simulink model "multiplier"  (Simulink 8.0)
settings: Solver=VariableStepDiscrete  StartTime=0.0  StopTime=50  RelTol=1e-3
settings Model: Creator=dell  LastModifiedBy=dell
settings DebuggingCC: FcnCallInpInsideContextMsg=EnableAllAsWarning

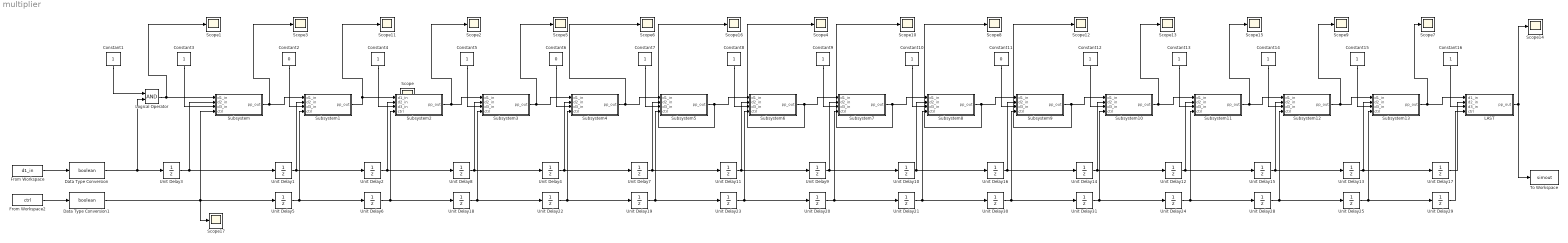
== system multiplier ==
  Constant{1,3..5,7..10,12..16} (13 alike) : Constant  OutDataTypeStr=boolean
  Constant11 : Constant  Value=0  OutDataTypeStr=boolean
  Constant2 : Constant  Value=0  OutDataTypeStr=boolean
  Constant6 : Constant  Value=0  OutDataTypeStr=boolean
  Data Type Conversion : DataTypeConversion  OutDataTypeStr=boolean
  Data Type Conversion1 : DataTypeConversion  OutDataTypeStr=boolean
  From Workspace : FromWorkspace  VariableName=d1_in  SampleTime=1
  From Workspace2 : FromWorkspace  VariableName=ctrl  SampleTime=1
  LAST : Subsystem
  Logical Operator : Logic  AllPortsSameDT=off  OutDataTypeStr=boolean
  Scope{,1..17} (18 alike) : Scope
      Scope10 settings: SaveName=ScopeData10
      Scope11 settings: SaveName=ScopeData11
      Scope12 settings: SaveName=ScopeData12
      Scope13 settings: SaveName=ScopeData13
      Scope14 settings: SaveName=ScopeData14
      Scope15 settings: SaveName=ScopeData15
      Scope16 settings: SaveName=ScopeData16
      Scope17 settings: SaveName=ScopeData17
      Scope2 settings: SaveName=ScopeData2
      Scope3 settings: SaveName=ScopeData3
      Scope4 settings: SaveName=ScopeData4
      Scope5 settings: SaveName=ScopeData5
      Scope6 settings: SaveName=ScopeData6
      Scope7 settings: SaveName=ScopeData7
      Scope8 settings: SaveName=ScopeData8
      Scope9 settings: SaveName=ScopeData9
  Subsystem : Subsystem
  Subsystem1 : Subsystem
  Subsystem10 : Subsystem
  Subsystem11 : Subsystem
  Subsystem12 : Subsystem
  Subsystem13 : Subsystem
  Subsystem2 : Subsystem
  Subsystem3 : Subsystem
  Subsystem4 : Subsystem
  Subsystem5 : Subsystem
  Subsystem6 : Subsystem
  Subsystem7 : Subsystem
  Subsystem8 : Subsystem
  Subsystem9 : Subsystem
  To Workspace : ToWorkspace  VariableName=simout  SampleTime=-1  SaveFormat=Timeseries
  Unit Delay{1..25,28..31} (29 alike) : UnitDelay
  wires:
  From Workspace/1 -> Data Type Conversion/1
  Logical Operator/1 -> Scope1/1, Subsystem/1(d1_in)
  Unit Delay3/1 -> Unit Delay1/1, Subsystem/2(d2_in)
  Subsystem/1(pp_out) -> Scope3/1, Subsystem1/1(d1_in)
  Subsystem1/1(pp_out) -> Scope11/1, Subsystem2/1(d1_in)
  Unit Delay5/1 -> Subsystem1/4(ctrl), Unit Delay6/1
  Constant1/1 -> Logical Operator/1
  Constant3/1 -> Subsystem/3(d3_in)
  Constant2/1 -> Subsystem1/3(d3_in)
  Constant4/1 -> Subsystem2/3(d3_in)
  From Workspace2/1 -> Data Type Conversion1/1
  Unit Delay1/1 -> Subsystem1/2(d2_in), Unit Delay2/1
  Unit Delay2/1 -> Subsystem2/2(d2_in), Unit Delay8/1
  Unit Delay8/1 -> Subsystem3/2(d2_in), Unit Delay4/1
  Unit Delay4/1 -> Subsystem4/2(d2_in), Unit Delay7/1
  Unit Delay7/1 -> Subsystem5/2(d2_in), Unit Delay11/1
  Unit Delay11/1 -> Subsystem6/2(d2_in), Unit Delay9/1
  Unit Delay9/1 -> Subsystem7/2(d2_in), Unit Delay10/1
  Unit Delay10/1 -> Subsystem8/2(d2_in), Unit Delay16/1
  Unit Delay16/1 -> Subsystem9/2(d2_in), Unit Delay14/1
  Unit Delay14/1 -> Subsystem10/2(d2_in), Unit Delay12/1
  Unit Delay12/1 -> Subsystem11/2(d2_in), Unit Delay15/1
  Unit Delay15/1 -> Subsystem12/2(d2_in), Unit Delay13/1
  Unit Delay13/1 -> Subsystem13/2(d2_in), Unit Delay17/1
  Unit Delay6/1 -> Subsystem2/4(ctrl), Unit Delay18/1
  Unit Delay18/1 -> Subsystem3/4(ctrl), Unit Delay22/1
  Unit Delay22/1 -> Subsystem4/4(ctrl), Unit Delay19/1
  Unit Delay19/1 -> Subsystem5/4(ctrl), Unit Delay23/1
  Unit Delay23/1 -> Subsystem6/4(ctrl), Unit Delay20/1
  Unit Delay20/1 -> Subsystem7/4(ctrl), Unit Delay21/1
  Unit Delay21/1 -> Subsystem8/4(ctrl), Unit Delay30/1
  Unit Delay30/1 -> Subsystem9/4(ctrl), Unit Delay31/1
  Unit Delay31/1 -> Subsystem10/4(ctrl), Unit Delay24/1
  Unit Delay24/1 -> Subsystem11/4(ctrl), Unit Delay28/1
  Unit Delay28/1 -> Subsystem12/4(ctrl), Unit Delay25/1
  Unit Delay25/1 -> Subsystem13/4(ctrl), Unit Delay29/1
  Subsystem2/1(pp_out) -> Scope2/1, Subsystem3/1(d1_in)
  Subsystem3/1(pp_out) -> Scope5/1, Subsystem4/1(d1_in)
  Subsystem4/1(pp_out) -> Scope6/1, Subsystem5/1(d1_in)
  Subsystem5/1(pp_out) -> Scope16/1, Subsystem6/1(d1_in)
  Subsystem6/1(pp_out) -> Scope4/1, Subsystem7/1(d1_in)
  Subsystem7/1(pp_out) -> Scope10/1, Subsystem8/1(d1_in)
  Subsystem8/1(pp_out) -> Scope8/1, Subsystem9/1(d1_in)
  Subsystem9/1(pp_out) -> Scope12/1, Subsystem10/1(d1_in)
  Subsystem10/1(pp_out) -> Scope13/1, Subsystem11/1(d1_in)
  Subsystem11/1(pp_out) -> Scope15/1, Subsystem12/1(d1_in)
  Subsystem12/1(pp_out) -> Scope9/1, Subsystem13/1(d1_in)
  Subsystem13/1(pp_out) -> Scope7/1, LAST/1(d1_in)
  Unit Delay17/1 -> LAST/2(d2_in)
  Unit Delay29/1 -> LAST/4(ctrl)
  Constant5/1 -> Subsystem3/3(d3_in)
  Constant6/1 -> Subsystem4/3(d3_in)
  Constant7/1 -> Subsystem5/3(d3_in)
  Constant8/1 -> Subsystem6/3(d3_in)
  Constant9/1 -> Subsystem7/3(d3_in)
  Constant10/1 -> Subsystem8/3(d3_in)
  Constant11/1 -> Subsystem9/3(d3_in)
  Constant12/1 -> Subsystem10/3(d3_in)
  Constant13/1 -> Subsystem11/3(d3_in)
  Constant14/1 -> Subsystem12/3(d3_in)
  Constant15/1 -> Subsystem13/3(d3_in)
  Constant16/1 -> LAST/3(d3_in)
  LAST/1(pp_out) -> Scope14/1, To Workspace/1
  Data Type Conversion/1 -> Logical Operator/2, Unit Delay3/1
  Data Type Conversion1/1 -> Scope17/1, Subsystem/4(ctrl), Unit Delay5/1

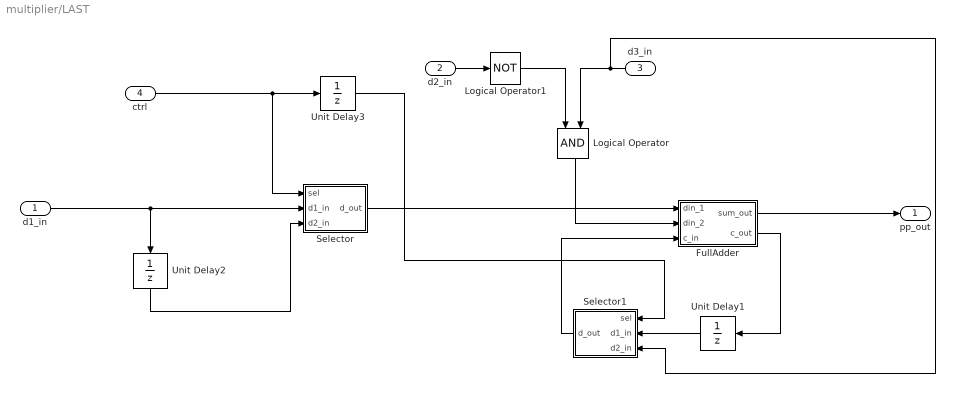
== system multiplier/LAST ==
  d1_in : Inport
  d2_in : Inport  Port=2
  d3_in : Inport  Port=3
  ctrl : Inport  Port=4
  FullAdder : Subsystem
  Logical Operator : Logic  AllPortsSameDT=off  OutDataTypeStr=boolean
  Logical Operator1 : Logic  Operator=NOT  AllPortsSameDT=off  OutDataTypeStr=boolean
  Selector : Subsystem
  Selector1 : Subsystem
  Unit Delay1 : UnitDelay
  Unit Delay2 : UnitDelay
  Unit Delay3 : UnitDelay
  pp_out : Outport
  wires:
  FullAdder/2(c_out) -> Unit Delay1/1
  d3_in/1 -> Logical Operator/2, Selector1/3(d2_in)
  ctrl/1 -> Unit Delay3/1, Selector/1(sel)
  d1_in/1 -> Selector/2(d1_in), Unit Delay2/1
  Unit Delay2/1 -> Selector/3(d2_in)
  d2_in/1 -> Logical Operator1/1
  Logical Operator/1 -> FullAdder/2(din_2)
  Selector/1(d_out) -> FullAdder/1(din_1)
  FullAdder/1(sum_out) -> pp_out/1
  Unit Delay1/1 -> Selector1/2(d1_in)
  Unit Delay3/1 -> Selector1/1(sel)
  Selector1/1(d_out) -> FullAdder/3(c_in)
  Logical Operator1/1 -> Logical Operator/1

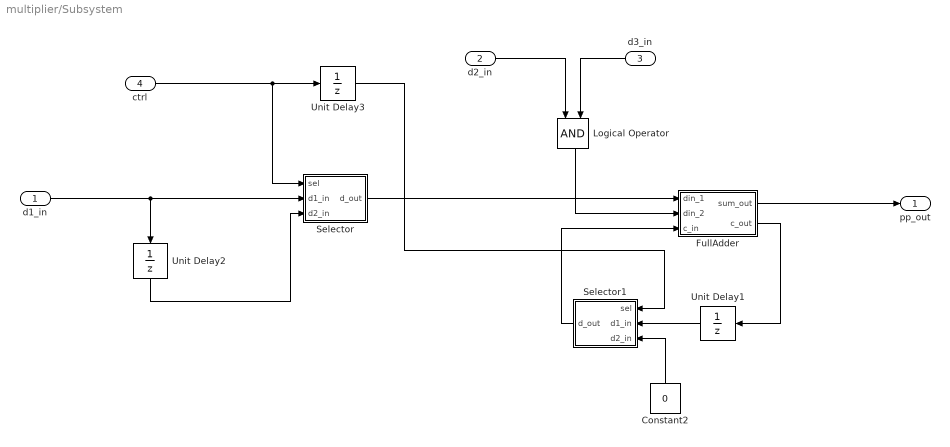
== system multiplier/Subsystem ==
  d1_in : Inport
  d2_in : Inport  Port=2
  d3_in : Inport  Port=3
  ctrl : Inport  Port=4
  Constant2 : Constant  Value=0  OutDataTypeStr=boolean
  FullAdder : Subsystem
  Logical Operator : Logic  AllPortsSameDT=off  OutDataTypeStr=boolean
  Selector : Subsystem
  Selector1 : Subsystem
  Unit Delay1 : UnitDelay
  Unit Delay2 : UnitDelay
  Unit Delay3 : UnitDelay
  pp_out : Outport
  wires:
  FullAdder/2(c_out) -> Unit Delay1/1
  d3_in/1 -> Logical Operator/2
  ctrl/1 -> Unit Delay3/1, Selector/1(sel)
  d1_in/1 -> Selector/2(d1_in), Unit Delay2/1
  Unit Delay2/1 -> Selector/3(d2_in)
  d2_in/1 -> Logical Operator/1
  Logical Operator/1 -> FullAdder/2(din_2)
  Selector/1(d_out) -> FullAdder/1(din_1)
  FullAdder/1(sum_out) -> pp_out/1
  Unit Delay1/1 -> Selector1/2(d1_in)
  Constant2/1 -> Selector1/3(d2_in)
  Unit Delay3/1 -> Selector1/1(sel)
  Selector1/1(d_out) -> FullAdder/3(c_in)

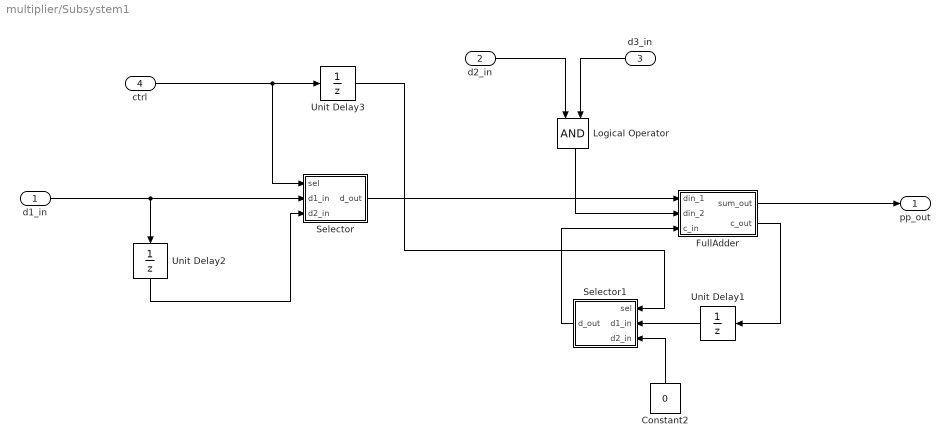
== system multiplier/Subsystem1 ==
  d1_in : Inport
  d2_in : Inport  Port=2
  d3_in : Inport  Port=3
  ctrl : Inport  Port=4
  Constant2 : Constant  Value=0  OutDataTypeStr=boolean
  FullAdder : Subsystem
  Logical Operator : Logic  AllPortsSameDT=off  OutDataTypeStr=boolean
  Selector : Subsystem
  Selector1 : Subsystem
  Unit Delay1 : UnitDelay
  Unit Delay2 : UnitDelay
  Unit Delay3 : UnitDelay
  pp_out : Outport
  wires:
  FullAdder/2(c_out) -> Unit Delay1/1
  d3_in/1 -> Logical Operator/2
  ctrl/1 -> Unit Delay3/1, Selector/1(sel)
  d1_in/1 -> Selector/2(d1_in), Unit Delay2/1
  Unit Delay2/1 -> Selector/3(d2_in)
  d2_in/1 -> Logical Operator/1
  Logical Operator/1 -> FullAdder/2(din_2)
  Selector/1(d_out) -> FullAdder/1(din_1)
  FullAdder/1(sum_out) -> pp_out/1
  Unit Delay1/1 -> Selector1/2(d1_in)
  Constant2/1 -> Selector1/3(d2_in)
  Unit Delay3/1 -> Selector1/1(sel)
  Selector1/1(d_out) -> FullAdder/3(c_in)

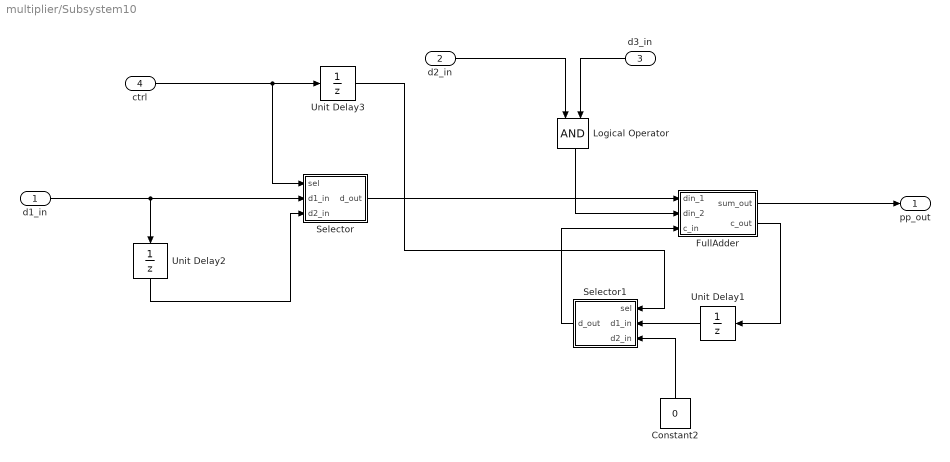
== system multiplier/Subsystem10 ==
  d1_in : Inport
  d2_in : Inport  Port=2
  d3_in : Inport  Port=3
  ctrl : Inport  Port=4
  Constant2 : Constant  Value=0  OutDataTypeStr=boolean
  FullAdder : Subsystem
  Logical Operator : Logic  AllPortsSameDT=off  OutDataTypeStr=boolean
  Selector : Subsystem
  Selector1 : Subsystem
  Unit Delay1 : UnitDelay
  Unit Delay2 : UnitDelay
  Unit Delay3 : UnitDelay
  pp_out : Outport
  wires:
  FullAdder/2(c_out) -> Unit Delay1/1
  d3_in/1 -> Logical Operator/2
  ctrl/1 -> Unit Delay3/1, Selector/1(sel)
  d1_in/1 -> Selector/2(d1_in), Unit Delay2/1
  Unit Delay2/1 -> Selector/3(d2_in)
  Logical Operator/1 -> FullAdder/2(din_2)
  Selector/1(d_out) -> FullAdder/1(din_1)
  FullAdder/1(sum_out) -> pp_out/1
  Unit Delay1/1 -> Selector1/2(d1_in)
  Unit Delay3/1 -> Selector1/1(sel)
  Selector1/1(d_out) -> FullAdder/3(c_in)
  d2_in/1 -> Logical Operator/1
  Constant2/1 -> Selector1/3(d2_in)

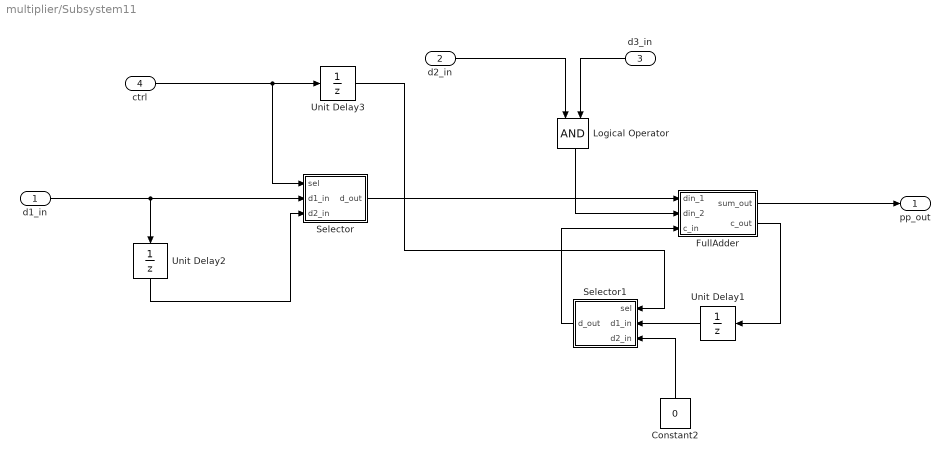
== system multiplier/Subsystem11 ==
  d1_in : Inport
  d2_in : Inport  Port=2
  d3_in : Inport  Port=3
  ctrl : Inport  Port=4
  Constant2 : Constant  Value=0  OutDataTypeStr=boolean
  FullAdder : Subsystem
  Logical Operator : Logic  AllPortsSameDT=off  OutDataTypeStr=boolean
  Selector : Subsystem
  Selector1 : Subsystem
  Unit Delay1 : UnitDelay
  Unit Delay2 : UnitDelay
  Unit Delay3 : UnitDelay
  pp_out : Outport
  wires:
  FullAdder/2(c_out) -> Unit Delay1/1
  d3_in/1 -> Logical Operator/2
  ctrl/1 -> Unit Delay3/1, Selector/1(sel)
  d1_in/1 -> Selector/2(d1_in), Unit Delay2/1
  Unit Delay2/1 -> Selector/3(d2_in)
  Logical Operator/1 -> FullAdder/2(din_2)
  Selector/1(d_out) -> FullAdder/1(din_1)
  FullAdder/1(sum_out) -> pp_out/1
  Unit Delay1/1 -> Selector1/2(d1_in)
  Unit Delay3/1 -> Selector1/1(sel)
  Selector1/1(d_out) -> FullAdder/3(c_in)
  d2_in/1 -> Logical Operator/1
  Constant2/1 -> Selector1/3(d2_in)

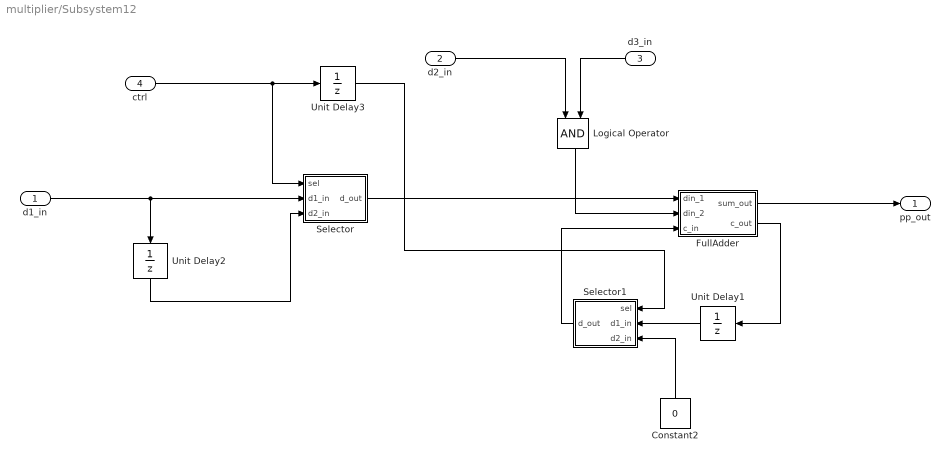
== system multiplier/Subsystem12 ==
  d1_in : Inport
  d2_in : Inport  Port=2
  d3_in : Inport  Port=3
  ctrl : Inport  Port=4
  Constant2 : Constant  Value=0  OutDataTypeStr=boolean
  FullAdder : Subsystem
  Logical Operator : Logic  AllPortsSameDT=off  OutDataTypeStr=boolean
  Selector : Subsystem
  Selector1 : Subsystem
  Unit Delay1 : UnitDelay
  Unit Delay2 : UnitDelay
  Unit Delay3 : UnitDelay
  pp_out : Outport
  wires:
  FullAdder/2(c_out) -> Unit Delay1/1
  d3_in/1 -> Logical Operator/2
  ctrl/1 -> Unit Delay3/1, Selector/1(sel)
  d1_in/1 -> Selector/2(d1_in), Unit Delay2/1
  Unit Delay2/1 -> Selector/3(d2_in)
  Logical Operator/1 -> FullAdder/2(din_2)
  Selector/1(d_out) -> FullAdder/1(din_1)
  FullAdder/1(sum_out) -> pp_out/1
  Unit Delay1/1 -> Selector1/2(d1_in)
  Unit Delay3/1 -> Selector1/1(sel)
  Selector1/1(d_out) -> FullAdder/3(c_in)
  d2_in/1 -> Logical Operator/1
  Constant2/1 -> Selector1/3(d2_in)

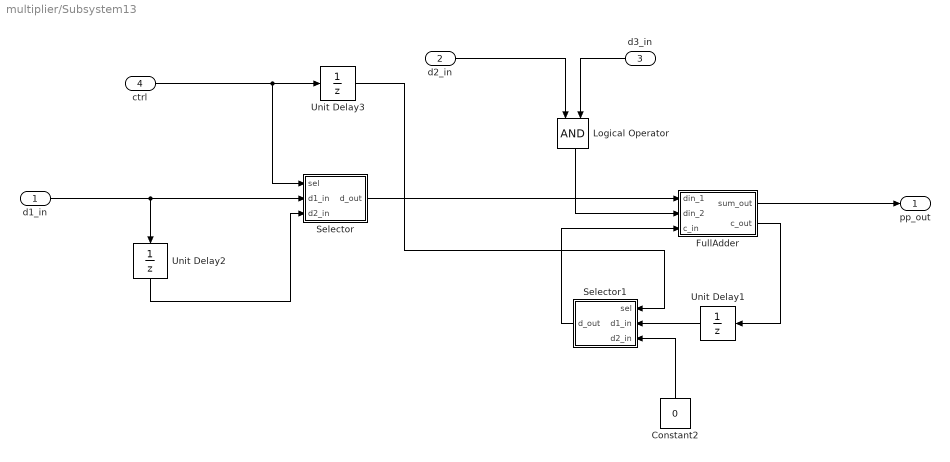
== system multiplier/Subsystem13 ==
  d1_in : Inport
  d2_in : Inport  Port=2
  d3_in : Inport  Port=3
  ctrl : Inport  Port=4
  Constant2 : Constant  Value=0  OutDataTypeStr=boolean
  FullAdder : Subsystem
  Logical Operator : Logic  AllPortsSameDT=off  OutDataTypeStr=boolean
  Selector : Subsystem
  Selector1 : Subsystem
  Unit Delay1 : UnitDelay
  Unit Delay2 : UnitDelay
  Unit Delay3 : UnitDelay
  pp_out : Outport
  wires:
  FullAdder/2(c_out) -> Unit Delay1/1
  d3_in/1 -> Logical Operator/2
  ctrl/1 -> Unit Delay3/1, Selector/1(sel)
  d1_in/1 -> Selector/2(d1_in), Unit Delay2/1
  Unit Delay2/1 -> Selector/3(d2_in)
  Logical Operator/1 -> FullAdder/2(din_2)
  Selector/1(d_out) -> FullAdder/1(din_1)
  FullAdder/1(sum_out) -> pp_out/1
  Unit Delay1/1 -> Selector1/2(d1_in)
  Unit Delay3/1 -> Selector1/1(sel)
  Selector1/1(d_out) -> FullAdder/3(c_in)
  d2_in/1 -> Logical Operator/1
  Constant2/1 -> Selector1/3(d2_in)

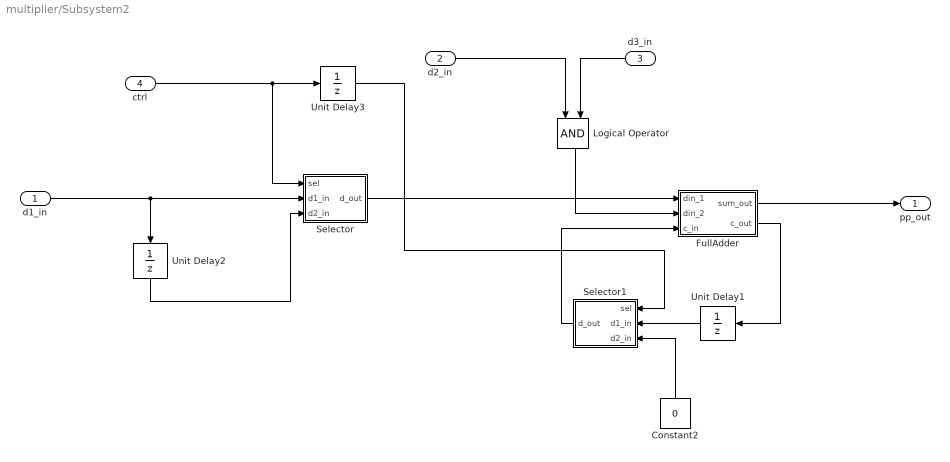
== system multiplier/Subsystem2 ==
  d1_in : Inport
  d2_in : Inport  Port=2
  d3_in : Inport  Port=3
  ctrl : Inport  Port=4
  Constant2 : Constant  Value=0  OutDataTypeStr=boolean
  FullAdder : Subsystem
  Logical Operator : Logic  AllPortsSameDT=off  OutDataTypeStr=boolean
  Selector : Subsystem
  Selector1 : Subsystem
  Unit Delay1 : UnitDelay
  Unit Delay2 : UnitDelay
  Unit Delay3 : UnitDelay
  pp_out : Outport
  wires:
  FullAdder/2(c_out) -> Unit Delay1/1
  d3_in/1 -> Logical Operator/2
  ctrl/1 -> Unit Delay3/1, Selector/1(sel)
  d1_in/1 -> Selector/2(d1_in), Unit Delay2/1
  Unit Delay2/1 -> Selector/3(d2_in)
  Logical Operator/1 -> FullAdder/2(din_2)
  Selector/1(d_out) -> FullAdder/1(din_1)
  FullAdder/1(sum_out) -> pp_out/1
  Unit Delay1/1 -> Selector1/2(d1_in)
  Unit Delay3/1 -> Selector1/1(sel)
  Selector1/1(d_out) -> FullAdder/3(c_in)
  d2_in/1 -> Logical Operator/1
  Constant2/1 -> Selector1/3(d2_in)

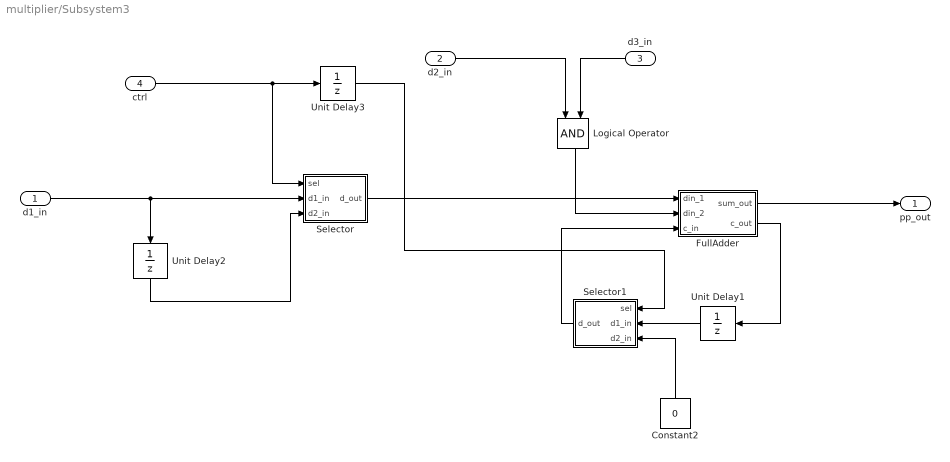
== system multiplier/Subsystem3 ==
  d1_in : Inport
  d2_in : Inport  Port=2
  d3_in : Inport  Port=3
  ctrl : Inport  Port=4
  Constant2 : Constant  Value=0  OutDataTypeStr=boolean
  FullAdder : Subsystem
  Logical Operator : Logic  AllPortsSameDT=off  OutDataTypeStr=boolean
  Selector : Subsystem
  Selector1 : Subsystem
  Unit Delay1 : UnitDelay
  Unit Delay2 : UnitDelay
  Unit Delay3 : UnitDelay
  pp_out : Outport
  wires:
  FullAdder/2(c_out) -> Unit Delay1/1
  d3_in/1 -> Logical Operator/2
  ctrl/1 -> Unit Delay3/1, Selector/1(sel)
  d1_in/1 -> Selector/2(d1_in), Unit Delay2/1
  Unit Delay2/1 -> Selector/3(d2_in)
  Logical Operator/1 -> FullAdder/2(din_2)
  Selector/1(d_out) -> FullAdder/1(din_1)
  FullAdder/1(sum_out) -> pp_out/1
  Unit Delay1/1 -> Selector1/2(d1_in)
  Unit Delay3/1 -> Selector1/1(sel)
  Selector1/1(d_out) -> FullAdder/3(c_in)
  d2_in/1 -> Logical Operator/1
  Constant2/1 -> Selector1/3(d2_in)

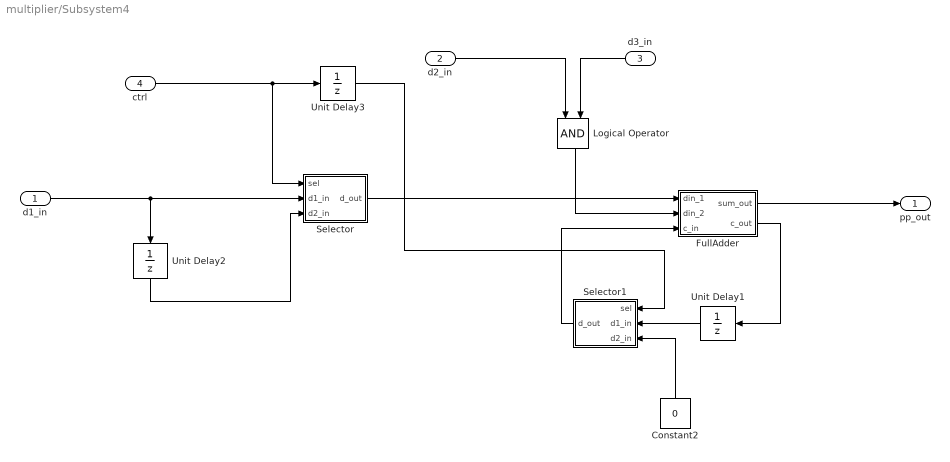
== system multiplier/Subsystem4 ==
  d1_in : Inport
  d2_in : Inport  Port=2
  d3_in : Inport  Port=3
  ctrl : Inport  Port=4
  Constant2 : Constant  Value=0  OutDataTypeStr=boolean
  FullAdder : Subsystem
  Logical Operator : Logic  AllPortsSameDT=off  OutDataTypeStr=boolean
  Selector : Subsystem
  Selector1 : Subsystem
  Unit Delay1 : UnitDelay
  Unit Delay2 : UnitDelay
  Unit Delay3 : UnitDelay
  pp_out : Outport
  wires:
  FullAdder/2(c_out) -> Unit Delay1/1
  d3_in/1 -> Logical Operator/2
  ctrl/1 -> Unit Delay3/1, Selector/1(sel)
  d1_in/1 -> Selector/2(d1_in), Unit Delay2/1
  Unit Delay2/1 -> Selector/3(d2_in)
  Logical Operator/1 -> FullAdder/2(din_2)
  Selector/1(d_out) -> FullAdder/1(din_1)
  FullAdder/1(sum_out) -> pp_out/1
  Unit Delay1/1 -> Selector1/2(d1_in)
  Unit Delay3/1 -> Selector1/1(sel)
  Selector1/1(d_out) -> FullAdder/3(c_in)
  d2_in/1 -> Logical Operator/1
  Constant2/1 -> Selector1/3(d2_in)

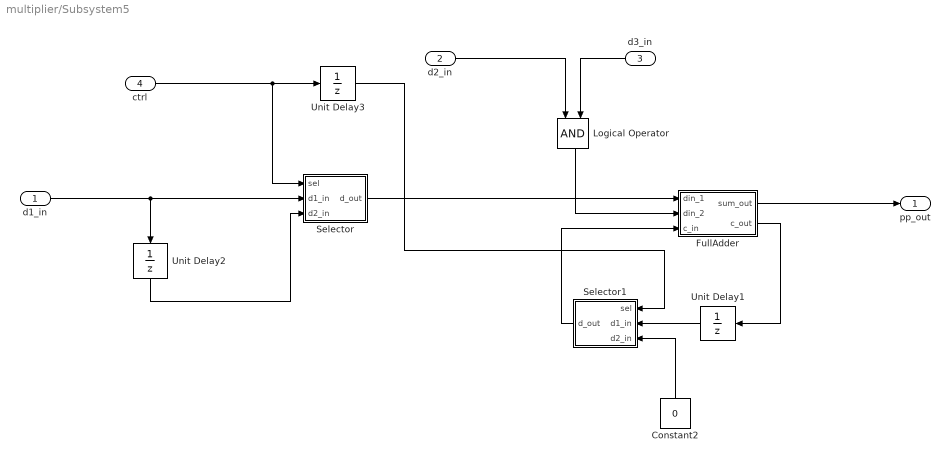
== system multiplier/Subsystem5 ==
  d1_in : Inport
  d2_in : Inport  Port=2
  d3_in : Inport  Port=3
  ctrl : Inport  Port=4
  Constant2 : Constant  Value=0  OutDataTypeStr=boolean
  FullAdder : Subsystem
  Logical Operator : Logic  AllPortsSameDT=off  OutDataTypeStr=boolean
  Selector : Subsystem
  Selector1 : Subsystem
  Unit Delay1 : UnitDelay
  Unit Delay2 : UnitDelay
  Unit Delay3 : UnitDelay
  pp_out : Outport
  wires:
  FullAdder/2(c_out) -> Unit Delay1/1
  d3_in/1 -> Logical Operator/2
  ctrl/1 -> Unit Delay3/1, Selector/1(sel)
  d1_in/1 -> Selector/2(d1_in), Unit Delay2/1
  Unit Delay2/1 -> Selector/3(d2_in)
  Logical Operator/1 -> FullAdder/2(din_2)
  Selector/1(d_out) -> FullAdder/1(din_1)
  FullAdder/1(sum_out) -> pp_out/1
  Unit Delay1/1 -> Selector1/2(d1_in)
  Unit Delay3/1 -> Selector1/1(sel)
  Selector1/1(d_out) -> FullAdder/3(c_in)
  d2_in/1 -> Logical Operator/1
  Constant2/1 -> Selector1/3(d2_in)

== system multiplier/Subsystem6 ==
  d1_in : Inport
  d2_in : Inport  Port=2
  d3_in : Inport  Port=3
  ctrl : Inport  Port=4
  Constant2 : Constant  Value=0  OutDataTypeStr=boolean
  FullAdder : Subsystem
  Logical Operator : Logic  AllPortsSameDT=off  OutDataTypeStr=boolean
  Selector : Subsystem
  Selector1 : Subsystem
  Unit Delay1 : UnitDelay
  Unit Delay2 : UnitDelay
  Unit Delay3 : UnitDelay
  pp_out : Outport
  wires:
  FullAdder/2(c_out) -> Unit Delay1/1
  d3_in/1 -> Logical Operator/2
  ctrl/1 -> Unit Delay3/1, Selector/1(sel)
  d1_in/1 -> Selector/2(d1_in), Unit Delay2/1
  Unit Delay2/1 -> Selector/3(d2_in)
  Logical Operator/1 -> FullAdder/2(din_2)
  Selector/1(d_out) -> FullAdder/1(din_1)
  FullAdder/1(sum_out) -> pp_out/1
  Unit Delay1/1 -> Selector1/2(d1_in)
  Unit Delay3/1 -> Selector1/1(sel)
  Selector1/1(d_out) -> FullAdder/3(c_in)
  d2_in/1 -> Logical Operator/1
  Constant2/1 -> Selector1/3(d2_in)

== system multiplier/Subsystem7 ==
  d1_in : Inport
  d2_in : Inport  Port=2
  d3_in : Inport  Port=3
  ctrl : Inport  Port=4
  Constant2 : Constant  Value=0  OutDataTypeStr=boolean
  FullAdder : Subsystem
  Logical Operator : Logic  AllPortsSameDT=off  OutDataTypeStr=boolean
  Selector : Subsystem
  Selector1 : Subsystem
  Unit Delay1 : UnitDelay
  Unit Delay2 : UnitDelay
  Unit Delay3 : UnitDelay
  pp_out : Outport
  wires:
  FullAdder/2(c_out) -> Unit Delay1/1
  d3_in/1 -> Logical Operator/2
  ctrl/1 -> Unit Delay3/1, Selector/1(sel)
  d1_in/1 -> Selector/2(d1_in), Unit Delay2/1
  Unit Delay2/1 -> Selector/3(d2_in)
  Logical Operator/1 -> FullAdder/2(din_2)
  Selector/1(d_out) -> FullAdder/1(din_1)
  FullAdder/1(sum_out) -> pp_out/1
  Unit Delay1/1 -> Selector1/2(d1_in)
  Unit Delay3/1 -> Selector1/1(sel)
  Selector1/1(d_out) -> FullAdder/3(c_in)
  d2_in/1 -> Logical Operator/1
  Constant2/1 -> Selector1/3(d2_in)

== system multiplier/Subsystem8 ==
  d1_in : Inport
  d2_in : Inport  Port=2
  d3_in : Inport  Port=3
  ctrl : Inport  Port=4
  Constant2 : Constant  Value=0  OutDataTypeStr=boolean
  FullAdder : Subsystem
  Logical Operator : Logic  AllPortsSameDT=off  OutDataTypeStr=boolean
  Selector : Subsystem
  Selector1 : Subsystem
  Unit Delay1 : UnitDelay
  Unit Delay2 : UnitDelay
  Unit Delay3 : UnitDelay
  pp_out : Outport
  wires:
  FullAdder/2(c_out) -> Unit Delay1/1
  d3_in/1 -> Logical Operator/2
  ctrl/1 -> Unit Delay3/1, Selector/1(sel)
  d1_in/1 -> Selector/2(d1_in), Unit Delay2/1
  Unit Delay2/1 -> Selector/3(d2_in)
  Logical Operator/1 -> FullAdder/2(din_2)
  Selector/1(d_out) -> FullAdder/1(din_1)
  FullAdder/1(sum_out) -> pp_out/1
  Unit Delay1/1 -> Selector1/2(d1_in)
  Unit Delay3/1 -> Selector1/1(sel)
  Selector1/1(d_out) -> FullAdder/3(c_in)
  d2_in/1 -> Logical Operator/1
  Constant2/1 -> Selector1/3(d2_in)

== system multiplier/Subsystem9 ==
  d1_in : Inport
  d2_in : Inport  Port=2
  d3_in : Inport  Port=3
  ctrl : Inport  Port=4
  Constant2 : Constant  Value=0  OutDataTypeStr=boolean
  FullAdder : Subsystem
  Logical Operator : Logic  AllPortsSameDT=off  OutDataTypeStr=boolean
  Selector : Subsystem
  Selector1 : Subsystem
  Unit Delay1 : UnitDelay
  Unit Delay2 : UnitDelay
  Unit Delay3 : UnitDelay
  pp_out : Outport
  wires:
  FullAdder/2(c_out) -> Unit Delay1/1
  d3_in/1 -> Logical Operator/2
  ctrl/1 -> Unit Delay3/1, Selector/1(sel)
  d1_in/1 -> Selector/2(d1_in), Unit Delay2/1
  Unit Delay2/1 -> Selector/3(d2_in)
  Logical Operator/1 -> FullAdder/2(din_2)
  Selector/1(d_out) -> FullAdder/1(din_1)
  FullAdder/1(sum_out) -> pp_out/1
  Unit Delay1/1 -> Selector1/2(d1_in)
  Unit Delay3/1 -> Selector1/1(sel)
  Selector1/1(d_out) -> FullAdder/3(c_in)
  d2_in/1 -> Logical Operator/1
  Constant2/1 -> Selector1/3(d2_in)

== system multiplier/LAST/FullAdder ==
  din_1 : Inport  OutDataTypeStr=boolean
  din_2 : Inport  Port=2  OutDataTypeStr=boolean
  c_in : Inport  Port=3  OutDataTypeStr=boolean
  Bus Creator : BusCreator  Inputs=3
  Combinatorial  Logic : CombinatorialLogic  TruthTable=[0;1;1;0;1;0;0;1]
  Combinatorial  Logic1 : CombinatorialLogic  TruthTable=[0;0;0;1;0;1;1;1]
  sum_out : Outport
  c_out : Outport  Port=2
  wires:
  Combinatorial  Logic/1 -> sum_out/1
  din_1/1 -> Bus Creator/1
  din_2/1 -> Bus Creator/2
  c_in/1 -> Bus Creator/3
  Bus Creator/1 -> Combinatorial  Logic/1, Combinatorial  Logic1/1
  Combinatorial  Logic1/1 -> c_out/1

== system multiplier/LAST/Selector ==
  sel : Inport
  d1_in : Inport  Port=2
  d2_in : Inport  Port=3
  Bus Creator : BusCreator  Inputs=3
  Combinatorial  Logic : CombinatorialLogic  TruthTable=[0;0;1;1;0;1;0;1]
  d_out : Outport
  wires:
  sel/1 -> Bus Creator/1
  d1_in/1 -> Bus Creator/2
  d2_in/1 -> Bus Creator/3
  Bus Creator/1 -> Combinatorial  Logic/1
  Combinatorial  Logic/1 -> d_out/1

== system multiplier/LAST/Selector1 ==
  sel : Inport
  d1_in : Inport  Port=2
  d2_in : Inport  Port=3
  Bus Creator : BusCreator  Inputs=3
  Combinatorial  Logic : CombinatorialLogic  TruthTable=[0;0;1;1;0;1;0;1]
  d_out : Outport
  wires:
  sel/1 -> Bus Creator/1
  d1_in/1 -> Bus Creator/2
  d2_in/1 -> Bus Creator/3
  Bus Creator/1 -> Combinatorial  Logic/1
  Combinatorial  Logic/1 -> d_out/1

== system multiplier/Subsystem/FullAdder ==
  din_1 : Inport  OutDataTypeStr=boolean
  din_2 : Inport  Port=2  OutDataTypeStr=boolean
  c_in : Inport  Port=3  OutDataTypeStr=boolean
  Bus Creator : BusCreator  Inputs=3
  Combinatorial  Logic : CombinatorialLogic  TruthTable=[0;1;1;0;1;0;0;1]
  Combinatorial  Logic1 : CombinatorialLogic  TruthTable=[0;0;0;1;0;1;1;1]
  sum_out : Outport
  c_out : Outport  Port=2
  wires:
  Combinatorial  Logic/1 -> sum_out/1
  din_1/1 -> Bus Creator/1
  din_2/1 -> Bus Creator/2
  c_in/1 -> Bus Creator/3
  Bus Creator/1 -> Combinatorial  Logic/1, Combinatorial  Logic1/1
  Combinatorial  Logic1/1 -> c_out/1

== system multiplier/Subsystem/Selector ==
  sel : Inport
  d1_in : Inport  Port=2
  d2_in : Inport  Port=3
  Bus Creator : BusCreator  Inputs=3
  Combinatorial  Logic : CombinatorialLogic  TruthTable=[0;0;1;1;0;1;0;1]
  d_out : Outport
  wires:
  sel/1 -> Bus Creator/1
  d1_in/1 -> Bus Creator/2
  d2_in/1 -> Bus Creator/3
  Bus Creator/1 -> Combinatorial  Logic/1
  Combinatorial  Logic/1 -> d_out/1

== system multiplier/Subsystem/Selector1 ==
  sel : Inport
  d1_in : Inport  Port=2
  d2_in : Inport  Port=3
  Bus Creator : BusCreator  Inputs=3
  Combinatorial  Logic : CombinatorialLogic  TruthTable=[0;0;1;1;0;1;0;1]
  d_out : Outport
  wires:
  sel/1 -> Bus Creator/1
  d1_in/1 -> Bus Creator/2
  d2_in/1 -> Bus Creator/3
  Bus Creator/1 -> Combinatorial  Logic/1
  Combinatorial  Logic/1 -> d_out/1

== system multiplier/Subsystem1/FullAdder ==
  din_1 : Inport  OutDataTypeStr=boolean
  din_2 : Inport  Port=2  OutDataTypeStr=boolean
  c_in : Inport  Port=3  OutDataTypeStr=boolean
  Bus Creator : BusCreator  Inputs=3
  Combinatorial  Logic : CombinatorialLogic  TruthTable=[0;1;1;0;1;0;0;1]
  Combinatorial  Logic1 : CombinatorialLogic  TruthTable=[0;0;0;1;0;1;1;1]
  sum_out : Outport
  c_out : Outport  Port=2
  wires:
  Combinatorial  Logic/1 -> sum_out/1
  din_1/1 -> Bus Creator/1
  din_2/1 -> Bus Creator/2
  c_in/1 -> Bus Creator/3
  Bus Creator/1 -> Combinatorial  Logic/1, Combinatorial  Logic1/1
  Combinatorial  Logic1/1 -> c_out/1

== system multiplier/Subsystem1/Selector ==
  sel : Inport
  d1_in : Inport  Port=2
  d2_in : Inport  Port=3
  Bus Creator : BusCreator  Inputs=3
  Combinatorial  Logic : CombinatorialLogic  TruthTable=[0;0;1;1;0;1;0;1]
  d_out : Outport
  wires:
  sel/1 -> Bus Creator/1
  d1_in/1 -> Bus Creator/2
  d2_in/1 -> Bus Creator/3
  Bus Creator/1 -> Combinatorial  Logic/1
  Combinatorial  Logic/1 -> d_out/1

== system multiplier/Subsystem1/Selector1 ==
  sel : Inport
  d1_in : Inport  Port=2
  d2_in : Inport  Port=3
  Bus Creator : BusCreator  Inputs=3
  Combinatorial  Logic : CombinatorialLogic  TruthTable=[0;0;1;1;0;1;0;1]
  d_out : Outport
  wires:
  sel/1 -> Bus Creator/1
  d1_in/1 -> Bus Creator/2
  d2_in/1 -> Bus Creator/3
  Bus Creator/1 -> Combinatorial  Logic/1
  Combinatorial  Logic/1 -> d_out/1

== system multiplier/Subsystem10/FullAdder ==
  din_1 : Inport  OutDataTypeStr=boolean
  din_2 : Inport  Port=2  OutDataTypeStr=boolean
  c_in : Inport  Port=3  OutDataTypeStr=boolean
  Bus Creator : BusCreator  Inputs=3
  Combinatorial  Logic : CombinatorialLogic  TruthTable=[0;1;1;0;1;0;0;1]
  Combinatorial  Logic1 : CombinatorialLogic  TruthTable=[0;0;0;1;0;1;1;1]
  sum_out : Outport
  c_out : Outport  Port=2
  wires:
  Combinatorial  Logic/1 -> sum_out/1
  din_1/1 -> Bus Creator/1
  din_2/1 -> Bus Creator/2
  c_in/1 -> Bus Creator/3
  Bus Creator/1 -> Combinatorial  Logic/1, Combinatorial  Logic1/1
  Combinatorial  Logic1/1 -> c_out/1

== system multiplier/Subsystem10/Selector ==
  sel : Inport
  d1_in : Inport  Port=2
  d2_in : Inport  Port=3
  Bus Creator : BusCreator  Inputs=3
  Combinatorial  Logic : CombinatorialLogic  TruthTable=[0;0;1;1;0;1;0;1]
  d_out : Outport
  wires:
  sel/1 -> Bus Creator/1
  d1_in/1 -> Bus Creator/2
  d2_in/1 -> Bus Creator/3
  Bus Creator/1 -> Combinatorial  Logic/1
  Combinatorial  Logic/1 -> d_out/1

== system multiplier/Subsystem10/Selector1 ==
  sel : Inport
  d1_in : Inport  Port=2
  d2_in : Inport  Port=3
  Bus Creator : BusCreator  Inputs=3
  Combinatorial  Logic : CombinatorialLogic  TruthTable=[0;0;1;1;0;1;0;1]
  d_out : Outport
  wires:
  sel/1 -> Bus Creator/1
  d1_in/1 -> Bus Creator/2
  d2_in/1 -> Bus Creator/3
  Bus Creator/1 -> Combinatorial  Logic/1
  Combinatorial  Logic/1 -> d_out/1

== system multiplier/Subsystem11/FullAdder ==
  din_1 : Inport  OutDataTypeStr=boolean
  din_2 : Inport  Port=2  OutDataTypeStr=boolean
  c_in : Inport  Port=3  OutDataTypeStr=boolean
  Bus Creator : BusCreator  Inputs=3
  Combinatorial  Logic : CombinatorialLogic  TruthTable=[0;1;1;0;1;0;0;1]
  Combinatorial  Logic1 : CombinatorialLogic  TruthTable=[0;0;0;1;0;1;1;1]
  sum_out : Outport
  c_out : Outport  Port=2
  wires:
  Combinatorial  Logic/1 -> sum_out/1
  din_1/1 -> Bus Creator/1
  din_2/1 -> Bus Creator/2
  c_in/1 -> Bus Creator/3
  Bus Creator/1 -> Combinatorial  Logic/1, Combinatorial  Logic1/1
  Combinatorial  Logic1/1 -> c_out/1

== system multiplier/Subsystem11/Selector ==
  sel : Inport
  d1_in : Inport  Port=2
  d2_in : Inport  Port=3
  Bus Creator : BusCreator  Inputs=3
  Combinatorial  Logic : CombinatorialLogic  TruthTable=[0;0;1;1;0;1;0;1]
  d_out : Outport
  wires:
  sel/1 -> Bus Creator/1
  d1_in/1 -> Bus Creator/2
  d2_in/1 -> Bus Creator/3
  Bus Creator/1 -> Combinatorial  Logic/1
  Combinatorial  Logic/1 -> d_out/1

== system multiplier/Subsystem11/Selector1 ==
  sel : Inport
  d1_in : Inport  Port=2
  d2_in : Inport  Port=3
  Bus Creator : BusCreator  Inputs=3
  Combinatorial  Logic : CombinatorialLogic  TruthTable=[0;0;1;1;0;1;0;1]
  d_out : Outport
  wires:
  sel/1 -> Bus Creator/1
  d1_in/1 -> Bus Creator/2
  d2_in/1 -> Bus Creator/3
  Bus Creator/1 -> Combinatorial  Logic/1
  Combinatorial  Logic/1 -> d_out/1

== system multiplier/Subsystem12/FullAdder ==
  din_1 : Inport  OutDataTypeStr=boolean
  din_2 : Inport  Port=2  OutDataTypeStr=boolean
  c_in : Inport  Port=3  OutDataTypeStr=boolean
  Bus Creator : BusCreator  Inputs=3
  Combinatorial  Logic : CombinatorialLogic  TruthTable=[0;1;1;0;1;0;0;1]
  Combinatorial  Logic1 : CombinatorialLogic  TruthTable=[0;0;0;1;0;1;1;1]
  sum_out : Outport
  c_out : Outport  Port=2
  wires:
  Combinatorial  Logic/1 -> sum_out/1
  din_1/1 -> Bus Creator/1
  din_2/1 -> Bus Creator/2
  c_in/1 -> Bus Creator/3
  Bus Creator/1 -> Combinatorial  Logic/1, Combinatorial  Logic1/1
  Combinatorial  Logic1/1 -> c_out/1

== system multiplier/Subsystem12/Selector ==
  sel : Inport
  d1_in : Inport  Port=2
  d2_in : Inport  Port=3
  Bus Creator : BusCreator  Inputs=3
  Combinatorial  Logic : CombinatorialLogic  TruthTable=[0;0;1;1;0;1;0;1]
  d_out : Outport
  wires:
  sel/1 -> Bus Creator/1
  d1_in/1 -> Bus Creator/2
  d2_in/1 -> Bus Creator/3
  Bus Creator/1 -> Combinatorial  Logic/1
  Combinatorial  Logic/1 -> d_out/1

== system multiplier/Subsystem12/Selector1 ==
  sel : Inport
  d1_in : Inport  Port=2
  d2_in : Inport  Port=3
  Bus Creator : BusCreator  Inputs=3
  Combinatorial  Logic : CombinatorialLogic  TruthTable=[0;0;1;1;0;1;0;1]
  d_out : Outport
  wires:
  sel/1 -> Bus Creator/1
  d1_in/1 -> Bus Creator/2
  d2_in/1 -> Bus Creator/3
  Bus Creator/1 -> Combinatorial  Logic/1
  Combinatorial  Logic/1 -> d_out/1

== system multiplier/Subsystem13/FullAdder ==
  din_1 : Inport  OutDataTypeStr=boolean
  din_2 : Inport  Port=2  OutDataTypeStr=boolean
  c_in : Inport  Port=3  OutDataTypeStr=boolean
  Bus Creator : BusCreator  Inputs=3
  Combinatorial  Logic : CombinatorialLogic  TruthTable=[0;1;1;0;1;0;0;1]
  Combinatorial  Logic1 : CombinatorialLogic  TruthTable=[0;0;0;1;0;1;1;1]
  sum_out : Outport
  c_out : Outport  Port=2
  wires:
  Combinatorial  Logic/1 -> sum_out/1
  din_1/1 -> Bus Creator/1
  din_2/1 -> Bus Creator/2
  c_in/1 -> Bus Creator/3
  Bus Creator/1 -> Combinatorial  Logic/1, Combinatorial  Logic1/1
  Combinatorial  Logic1/1 -> c_out/1

== system multiplier/Subsystem13/Selector ==
  sel : Inport
  d1_in : Inport  Port=2
  d2_in : Inport  Port=3
  Bus Creator : BusCreator  Inputs=3
  Combinatorial  Logic : CombinatorialLogic  TruthTable=[0;0;1;1;0;1;0;1]
  d_out : Outport
  wires:
  sel/1 -> Bus Creator/1
  d1_in/1 -> Bus Creator/2
  d2_in/1 -> Bus Creator/3
  Bus Creator/1 -> Combinatorial  Logic/1
  Combinatorial  Logic/1 -> d_out/1

== system multiplier/Subsystem13/Selector1 ==
  sel : Inport
  d1_in : Inport  Port=2
  d2_in : Inport  Port=3
  Bus Creator : BusCreator  Inputs=3
  Combinatorial  Logic : CombinatorialLogic  TruthTable=[0;0;1;1;0;1;0;1]
  d_out : Outport
  wires:
  sel/1 -> Bus Creator/1
  d1_in/1 -> Bus Creator/2
  d2_in/1 -> Bus Creator/3
  Bus Creator/1 -> Combinatorial  Logic/1
  Combinatorial  Logic/1 -> d_out/1

== system multiplier/Subsystem2/FullAdder ==
  din_1 : Inport  OutDataTypeStr=boolean
  din_2 : Inport  Port=2  OutDataTypeStr=boolean
  c_in : Inport  Port=3  OutDataTypeStr=boolean
  Bus Creator : BusCreator  Inputs=3
  Combinatorial  Logic : CombinatorialLogic  TruthTable=[0;1;1;0;1;0;0;1]
  Combinatorial  Logic1 : CombinatorialLogic  TruthTable=[0;0;0;1;0;1;1;1]
  sum_out : Outport
  c_out : Outport  Port=2
  wires:
  Combinatorial  Logic/1 -> sum_out/1
  din_1/1 -> Bus Creator/1
  din_2/1 -> Bus Creator/2
  c_in/1 -> Bus Creator/3
  Bus Creator/1 -> Combinatorial  Logic/1, Combinatorial  Logic1/1
  Combinatorial  Logic1/1 -> c_out/1

== system multiplier/Subsystem2/Selector ==
  sel : Inport
  d1_in : Inport  Port=2
  d2_in : Inport  Port=3
  Bus Creator : BusCreator  Inputs=3
  Combinatorial  Logic : CombinatorialLogic  TruthTable=[0;0;1;1;0;1;0;1]
  d_out : Outport
  wires:
  sel/1 -> Bus Creator/1
  d1_in/1 -> Bus Creator/2
  d2_in/1 -> Bus Creator/3
  Bus Creator/1 -> Combinatorial  Logic/1
  Combinatorial  Logic/1 -> d_out/1

== system multiplier/Subsystem2/Selector1 ==
  sel : Inport
  d1_in : Inport  Port=2
  d2_in : Inport  Port=3
  Bus Creator : BusCreator  Inputs=3
  Combinatorial  Logic : CombinatorialLogic  TruthTable=[0;0;1;1;0;1;0;1]
  d_out : Outport
  wires:
  sel/1 -> Bus Creator/1
  d1_in/1 -> Bus Creator/2
  d2_in/1 -> Bus Creator/3
  Bus Creator/1 -> Combinatorial  Logic/1
  Combinatorial  Logic/1 -> d_out/1

== system multiplier/Subsystem3/FullAdder ==
  din_1 : Inport  OutDataTypeStr=boolean
  din_2 : Inport  Port=2  OutDataTypeStr=boolean
  c_in : Inport  Port=3  OutDataTypeStr=boolean
  Bus Creator : BusCreator  Inputs=3
  Combinatorial  Logic : CombinatorialLogic  TruthTable=[0;1;1;0;1;0;0;1]
  Combinatorial  Logic1 : CombinatorialLogic  TruthTable=[0;0;0;1;0;1;1;1]
  sum_out : Outport
  c_out : Outport  Port=2
  wires:
  Combinatorial  Logic/1 -> sum_out/1
  din_1/1 -> Bus Creator/1
  din_2/1 -> Bus Creator/2
  c_in/1 -> Bus Creator/3
  Bus Creator/1 -> Combinatorial  Logic/1, Combinatorial  Logic1/1
  Combinatorial  Logic1/1 -> c_out/1

== system multiplier/Subsystem3/Selector ==
  sel : Inport
  d1_in : Inport  Port=2
  d2_in : Inport  Port=3
  Bus Creator : BusCreator  Inputs=3
  Combinatorial  Logic : CombinatorialLogic  TruthTable=[0;0;1;1;0;1;0;1]
  d_out : Outport
  wires:
  sel/1 -> Bus Creator/1
  d1_in/1 -> Bus Creator/2
  d2_in/1 -> Bus Creator/3
  Bus Creator/1 -> Combinatorial  Logic/1
  Combinatorial  Logic/1 -> d_out/1

== system multiplier/Subsystem3/Selector1 ==
  sel : Inport
  d1_in : Inport  Port=2
  d2_in : Inport  Port=3
  Bus Creator : BusCreator  Inputs=3
  Combinatorial  Logic : CombinatorialLogic  TruthTable=[0;0;1;1;0;1;0;1]
  d_out : Outport
  wires:
  sel/1 -> Bus Creator/1
  d1_in/1 -> Bus Creator/2
  d2_in/1 -> Bus Creator/3
  Bus Creator/1 -> Combinatorial  Logic/1
  Combinatorial  Logic/1 -> d_out/1

== system multiplier/Subsystem4/FullAdder ==
  din_1 : Inport  OutDataTypeStr=boolean
  din_2 : Inport  Port=2  OutDataTypeStr=boolean
  c_in : Inport  Port=3  OutDataTypeStr=boolean
  Bus Creator : BusCreator  Inputs=3
  Combinatorial  Logic : CombinatorialLogic  TruthTable=[0;1;1;0;1;0;0;1]
  Combinatorial  Logic1 : CombinatorialLogic  TruthTable=[0;0;0;1;0;1;1;1]
  sum_out : Outport
  c_out : Outport  Port=2
  wires:
  Combinatorial  Logic/1 -> sum_out/1
  din_1/1 -> Bus Creator/1
  din_2/1 -> Bus Creator/2
  c_in/1 -> Bus Creator/3
  Bus Creator/1 -> Combinatorial  Logic/1, Combinatorial  Logic1/1
  Combinatorial  Logic1/1 -> c_out/1

== system multiplier/Subsystem4/Selector ==
  sel : Inport
  d1_in : Inport  Port=2
  d2_in : Inport  Port=3
  Bus Creator : BusCreator  Inputs=3
  Combinatorial  Logic : CombinatorialLogic  TruthTable=[0;0;1;1;0;1;0;1]
  d_out : Outport
  wires:
  sel/1 -> Bus Creator/1
  d1_in/1 -> Bus Creator/2
  d2_in/1 -> Bus Creator/3
  Bus Creator/1 -> Combinatorial  Logic/1
  Combinatorial  Logic/1 -> d_out/1

== system multiplier/Subsystem4/Selector1 ==
  sel : Inport
  d1_in : Inport  Port=2
  d2_in : Inport  Port=3
  Bus Creator : BusCreator  Inputs=3
  Combinatorial  Logic : CombinatorialLogic  TruthTable=[0;0;1;1;0;1;0;1]
  d_out : Outport
  wires:
  sel/1 -> Bus Creator/1
  d1_in/1 -> Bus Creator/2
  d2_in/1 -> Bus Creator/3
  Bus Creator/1 -> Combinatorial  Logic/1
  Combinatorial  Logic/1 -> d_out/1

== system multiplier/Subsystem5/FullAdder ==
  din_1 : Inport  OutDataTypeStr=boolean
  din_2 : Inport  Port=2  OutDataTypeStr=boolean
  c_in : Inport  Port=3  OutDataTypeStr=boolean
  Bus Creator : BusCreator  Inputs=3
  Combinatorial  Logic : CombinatorialLogic  TruthTable=[0;1;1;0;1;0;0;1]
  Combinatorial  Logic1 : CombinatorialLogic  TruthTable=[0;0;0;1;0;1;1;1]
  sum_out : Outport
  c_out : Outport  Port=2
  wires:
  Combinatorial  Logic/1 -> sum_out/1
  din_1/1 -> Bus Creator/1
  din_2/1 -> Bus Creator/2
  c_in/1 -> Bus Creator/3
  Bus Creator/1 -> Combinatorial  Logic/1, Combinatorial  Logic1/1
  Combinatorial  Logic1/1 -> c_out/1

== system multiplier/Subsystem5/Selector ==
  sel : Inport
  d1_in : Inport  Port=2
  d2_in : Inport  Port=3
  Bus Creator : BusCreator  Inputs=3
  Combinatorial  Logic : CombinatorialLogic  TruthTable=[0;0;1;1;0;1;0;1]
  d_out : Outport
  wires:
  sel/1 -> Bus Creator/1
  d1_in/1 -> Bus Creator/2
  d2_in/1 -> Bus Creator/3
  Bus Creator/1 -> Combinatorial  Logic/1
  Combinatorial  Logic/1 -> d_out/1

== system multiplier/Subsystem5/Selector1 ==
  sel : Inport
  d1_in : Inport  Port=2
  d2_in : Inport  Port=3
  Bus Creator : BusCreator  Inputs=3
  Combinatorial  Logic : CombinatorialLogic  TruthTable=[0;0;1;1;0;1;0;1]
  d_out : Outport
  wires:
  sel/1 -> Bus Creator/1
  d1_in/1 -> Bus Creator/2
  d2_in/1 -> Bus Creator/3
  Bus Creator/1 -> Combinatorial  Logic/1
  Combinatorial  Logic/1 -> d_out/1

== system multiplier/Subsystem6/FullAdder ==
  din_1 : Inport  OutDataTypeStr=boolean
  din_2 : Inport  Port=2  OutDataTypeStr=boolean
  c_in : Inport  Port=3  OutDataTypeStr=boolean
  Bus Creator : BusCreator  Inputs=3
  Combinatorial  Logic : CombinatorialLogic  TruthTable=[0;1;1;0;1;0;0;1]
  Combinatorial  Logic1 : CombinatorialLogic  TruthTable=[0;0;0;1;0;1;1;1]
  sum_out : Outport
  c_out : Outport  Port=2
  wires:
  Combinatorial  Logic/1 -> sum_out/1
  din_1/1 -> Bus Creator/1
  din_2/1 -> Bus Creator/2
  c_in/1 -> Bus Creator/3
  Bus Creator/1 -> Combinatorial  Logic/1, Combinatorial  Logic1/1
  Combinatorial  Logic1/1 -> c_out/1

== system multiplier/Subsystem6/Selector ==
  sel : Inport
  d1_in : Inport  Port=2
  d2_in : Inport  Port=3
  Bus Creator : BusCreator  Inputs=3
  Combinatorial  Logic : CombinatorialLogic  TruthTable=[0;0;1;1;0;1;0;1]
  d_out : Outport
  wires:
  sel/1 -> Bus Creator/1
  d1_in/1 -> Bus Creator/2
  d2_in/1 -> Bus Creator/3
  Bus Creator/1 -> Combinatorial  Logic/1
  Combinatorial  Logic/1 -> d_out/1

== system multiplier/Subsystem6/Selector1 ==
  sel : Inport
  d1_in : Inport  Port=2
  d2_in : Inport  Port=3
  Bus Creator : BusCreator  Inputs=3
  Combinatorial  Logic : CombinatorialLogic  TruthTable=[0;0;1;1;0;1;0;1]
  d_out : Outport
  wires:
  sel/1 -> Bus Creator/1
  d1_in/1 -> Bus Creator/2
  d2_in/1 -> Bus Creator/3
  Bus Creator/1 -> Combinatorial  Logic/1
  Combinatorial  Logic/1 -> d_out/1

== system multiplier/Subsystem7/FullAdder ==
  din_1 : Inport  OutDataTypeStr=boolean
  din_2 : Inport  Port=2  OutDataTypeStr=boolean
  c_in : Inport  Port=3  OutDataTypeStr=boolean
  Bus Creator : BusCreator  Inputs=3
  Combinatorial  Logic : CombinatorialLogic  TruthTable=[0;1;1;0;1;0;0;1]
  Combinatorial  Logic1 : CombinatorialLogic  TruthTable=[0;0;0;1;0;1;1;1]
  sum_out : Outport
  c_out : Outport  Port=2
  wires:
  Combinatorial  Logic/1 -> sum_out/1
  din_1/1 -> Bus Creator/1
  din_2/1 -> Bus Creator/2
  c_in/1 -> Bus Creator/3
  Bus Creator/1 -> Combinatorial  Logic/1, Combinatorial  Logic1/1
  Combinatorial  Logic1/1 -> c_out/1

== system multiplier/Subsystem7/Selector ==
  sel : Inport
  d1_in : Inport  Port=2
  d2_in : Inport  Port=3
  Bus Creator : BusCreator  Inputs=3
  Combinatorial  Logic : CombinatorialLogic  TruthTable=[0;0;1;1;0;1;0;1]
  d_out : Outport
  wires:
  sel/1 -> Bus Creator/1
  d1_in/1 -> Bus Creator/2
  d2_in/1 -> Bus Creator/3
  Bus Creator/1 -> Combinatorial  Logic/1
  Combinatorial  Logic/1 -> d_out/1

== system multiplier/Subsystem7/Selector1 ==
  sel : Inport
  d1_in : Inport  Port=2
  d2_in : Inport  Port=3
  Bus Creator : BusCreator  Inputs=3
  Combinatorial  Logic : CombinatorialLogic  TruthTable=[0;0;1;1;0;1;0;1]
  d_out : Outport
  wires:
  sel/1 -> Bus Creator/1
  d1_in/1 -> Bus Creator/2
  d2_in/1 -> Bus Creator/3
  Bus Creator/1 -> Combinatorial  Logic/1
  Combinatorial  Logic/1 -> d_out/1

== system multiplier/Subsystem8/FullAdder ==
  din_1 : Inport  OutDataTypeStr=boolean
  din_2 : Inport  Port=2  OutDataTypeStr=boolean
  c_in : Inport  Port=3  OutDataTypeStr=boolean
  Bus Creator : BusCreator  Inputs=3
  Combinatorial  Logic : CombinatorialLogic  TruthTable=[0;1;1;0;1;0;0;1]
  Combinatorial  Logic1 : CombinatorialLogic  TruthTable=[0;0;0;1;0;1;1;1]
  sum_out : Outport
  c_out : Outport  Port=2
  wires:
  Combinatorial  Logic/1 -> sum_out/1
  din_1/1 -> Bus Creator/1
  din_2/1 -> Bus Creator/2
  c_in/1 -> Bus Creator/3
  Bus Creator/1 -> Combinatorial  Logic/1, Combinatorial  Logic1/1
  Combinatorial  Logic1/1 -> c_out/1

== system multiplier/Subsystem8/Selector ==
  sel : Inport
  d1_in : Inport  Port=2
  d2_in : Inport  Port=3
  Bus Creator : BusCreator  Inputs=3
  Combinatorial  Logic : CombinatorialLogic  TruthTable=[0;0;1;1;0;1;0;1]
  d_out : Outport
  wires:
  sel/1 -> Bus Creator/1
  d1_in/1 -> Bus Creator/2
  d2_in/1 -> Bus Creator/3
  Bus Creator/1 -> Combinatorial  Logic/1
  Combinatorial  Logic/1 -> d_out/1

== system multiplier/Subsystem8/Selector1 ==
  sel : Inport
  d1_in : Inport  Port=2
  d2_in : Inport  Port=3
  Bus Creator : BusCreator  Inputs=3
  Combinatorial  Logic : CombinatorialLogic  TruthTable=[0;0;1;1;0;1;0;1]
  d_out : Outport
  wires:
  sel/1 -> Bus Creator/1
  d1_in/1 -> Bus Creator/2
  d2_in/1 -> Bus Creator/3
  Bus Creator/1 -> Combinatorial  Logic/1
  Combinatorial  Logic/1 -> d_out/1

== system multiplier/Subsystem9/FullAdder ==
  din_1 : Inport  OutDataTypeStr=boolean
  din_2 : Inport  Port=2  OutDataTypeStr=boolean
  c_in : Inport  Port=3  OutDataTypeStr=boolean
  Bus Creator : BusCreator  Inputs=3
  Combinatorial  Logic : CombinatorialLogic  TruthTable=[0;1;1;0;1;0;0;1]
  Combinatorial  Logic1 : CombinatorialLogic  TruthTable=[0;0;0;1;0;1;1;1]
  sum_out : Outport
  c_out : Outport  Port=2
  wires:
  Combinatorial  Logic/1 -> sum_out/1
  din_1/1 -> Bus Creator/1
  din_2/1 -> Bus Creator/2
  c_in/1 -> Bus Creator/3
  Bus Creator/1 -> Combinatorial  Logic/1, Combinatorial  Logic1/1
  Combinatorial  Logic1/1 -> c_out/1

== system multiplier/Subsystem9/Selector ==
  sel : Inport
  d1_in : Inport  Port=2
  d2_in : Inport  Port=3
  Bus Creator : BusCreator  Inputs=3
  Combinatorial  Logic : CombinatorialLogic  TruthTable=[0;0;1;1;0;1;0;1]
  d_out : Outport
  wires:
  sel/1 -> Bus Creator/1
  d1_in/1 -> Bus Creator/2
  d2_in/1 -> Bus Creator/3
  Bus Creator/1 -> Combinatorial  Logic/1
  Combinatorial  Logic/1 -> d_out/1

== system multiplier/Subsystem9/Selector1 ==
  sel : Inport
  d1_in : Inport  Port=2
  d2_in : Inport  Port=3
  Bus Creator : BusCreator  Inputs=3
  Combinatorial  Logic : CombinatorialLogic  TruthTable=[0;0;1;1;0;1;0;1]
  d_out : Outport
  wires:
  sel/1 -> Bus Creator/1
  d1_in/1 -> Bus Creator/2
  d2_in/1 -> Bus Creator/3
  Bus Creator/1 -> Combinatorial  Logic/1
  Combinatorial  Logic/1 -> d_out/1
